simulink model "Concave_hipp"  (R2023a)
settings: Solver=ode3  StartTime=0.0  StopTime=100  FixedStep=0.0001  RelTol=1e-3
values from neighbouring files (symbols this model uses):
  d_pitch_2 = 1    [simulation_para.m]
  d_roll_2 = 1    [simulation_para.m]
  d_yaw_2 = 1    [simulation_para.m]
  disturbance = 0    [simulation_para.m]
  dpitch_para = [1,1,1,0.01]    [simulation_para.m]
  droll_para = [1,1,1,0.01]    [simulation_para.m]
  dyaw_para = [1,1,1,0.01]    [simulation_para.m]
  k_pos_2 = 8    [simulation_para.m]
  k_vel_2 = 8    [simulation_para.m]
  kp_para = [8,20,1,0.01]    [simulation_para.m]
  kv_para = [8,20,1,0.01]    [simulation_para.m]
  p_pitch_2 = 10    [simulation_para.m]
  p_roll_2 = 10    [simulation_para.m]
  p_yaw_2 = 10    [simulation_para.m]
  ppitch_para = [10,10,1,0.01]    [simulation_para.m]
  proll_para = [10,10,1,0.01]    [simulation_para.m]
  pyaw_para = [10,20,1,0.01]    [simulation_para.m]
  Q1 = -8    [simulation_para.m]
  Q2 = -10    [simulation_para.m]
  Q3 = -[0.01,5,8]    [simulation_para.m]
  Q4 = -[0.001,0.1,0.1]    [simulation_para.m]
  Qc1 = -[8,50,1,0.01]    [simulation_para.m]
  Qc2 = -[10,80,1,0.02]    [simulation_para.m]
  Qc3 = [qc3_1;qc3_2;qc3_3]    [simulation_para.m]
  Qc4 = [qc4_1;qc4_2;qc4_3]    [simulation_para.m]
(part 2 of 2)

== matlab function Concave_hipp/PDController/Geo Controller1 ==
  data: r input; x input; tau output; p_roll input; p_pitch input; p_yaw input; d_roll input; d_pitch input; d_yaw input
function tau = fcn(r, x,p_roll,p_pitch,p_yaw,d_roll,d_pitch,d_yaw)
%% Geo Controller following
% D. Mellinger and V. Kumar. Minimum Snap Trajectory Generation and Control
% for Quadrotors. ICRA, 2011
% D.A. Duecker,  A. Hackbarth, T. Johannink, E. Kreuzer, and E. Solowjow. 
% Micro Underwater Vehicle Hydrobatics: A Submerged Furuta Pendulum. ICRA,
% 2018.
%

% Gains that work for backup
% p_roll  = 4;
% p_pitch = 4;
% p_yaw   = 4;
% 
% d_roll  = 1.5;
% d_pitch = 2;
% d_yaw   = 2;

K_p = diag([p_roll, p_pitch, p_yaw]);
K_d = diag([d_roll, d_pitch, d_yaw]);

%% Transform attitude into SO(3)
Phi     = x(1:3);
Phi_des = r(1:3);

R       = R_euler(Phi);
R_des   = R_euler(Phi_des);

%% Compute control errors

% Compute attitude error on SO(3)
e_R = 0.5*(R_des'*R - R'*R_des);

% Extract the skew-symmetric part of the rotation error matrix as a vector
e_R_vec = [e_R(3,2); e_R(1,3); e_R(2,1)]; 

% Compute the error in the angular velocities
omega     = x(4:6);
K_omega = diag([1,2,2]);
omega_des = K_omega * (Phi_des-Phi);
e_omega   = omega - omega_des;

%% Compute controller output
% Apply gains given as parameters
tau = - K_p * e_R_vec - K_d * e_omega;

end

function R = R_euler(Phi)
%R_EULER Function that maps the Z-Y-X Euler angles to the corresponding
%rotation matrix

phi = Phi(1); theta = Phi(2); psi = Phi(3);

R = [  cos(psi)*cos(theta)  cos(psi)*sin(theta)*sin(phi)-sin(psi)*cos(phi)  cos(psi)*cos(phi)*sin(theta)+sin(psi)*sin(phi) ;
       sin(psi)*cos(theta)  sin(psi)*sin(theta)*sin(phi)+cos(psi)*cos(phi)  sin(psi)*cos(phi)*sin(theta)-cos(psi)*sin(phi) ;
      -sin(theta)           cos(theta)*sin(phi)                             cos(theta)*cos(phi)                            ];
end

== matlab function Concave_hipp/PDController/MATLAB Function1 ==
  data: theta_des input; theta_des output; x input
function theta_des = fcn(theta_des, x)
yaw = x(6);
yaw_des = theta_des(3);
e_yaw = yaw_des-yaw;

% jump from -pi to +pi
if (e_yaw > pi)
    yaw_des = yaw_des - 2*pi;
% jump from +pi to -pi
elseif (-e_yaw > pi)
    yaw_des = yaw_des + 2*pi;
end
theta_des(3) = yaw_des;
